simulink model "ELEC4110"  (Simulink 10.1)
settings: Solver=FixedStepDiscrete  StartTime=0.0  StopTime=200  RelTol=1e-3
PreLoadFcn:
  | qpsktxrx = commqpsktxrx_init();
InitFcn:
  | %qpsktxrx = commqpsktxrx_init();
  | ELEC4110_Init;
values from neighbouring files (symbols this model uses):
  H_CSIR = H_static    [ELEC4110_Init.m]
  maxTOffset = 50    [ELEC4110_Init.m]
  numInterpRx = 8    [ELEC4110_Init.m]
  numSampPerSym = RxSampleSize / TotalFrameSize    [ELEC4110_Init.m]
  PreambleSize = losmimo.SeqLength    [ELEC4110_Init.m]
  TotalDataPreambleSize = losmimo.DataLength/log2(losmimo.M) + losmimo.SeqLength    [ELEC4110_Init.m]
  TxPreamble = [losmimo.PNSymbols; losmimo.PNSymbols1; losmimo.PNSymbols2; losmimo.PNSymbols3; losmimo.PNSymbols4; losmimo.PNSymbols5; losmimo.PNSymbols6; losmimo.PNSymbols7]    [ELEC4110_Init.m]
undefined symbols (not defined in the file or in its folder): losmimo
libraries: commfilt2 x4, commsink2 x2, commdigbbndam3 x2, commchan3 x1, dspsrcs4 x1, dspsigops x1
Description:
  | QPSK Transmitter and Receiver.
  | 
  | This model shows the implementation of a QPSK transmitter and receiver.
settings Model: FPTRunName=Active  Creator=The MathWorks, Inc.  LastModifiedBy=eeknlau
settings DataIOCC: LimitDataPoints=on  SaveOutput=off  SaveTime=off
settings OptimizationCC: BooleanDataType=off  DefaultParameterBehavior=Inlined  ExpressionDepthLimit=2147483647  LocalBlockOutputs=off
settings DebuggingCC: AlgebraicLoopMsg=error  SolverPrmCheckMsg=warning  SingleTaskRateTransMsg=error  ParameterPrecisionLossMsg=none  AllowSymbolicDim=off  StateNameClashWarn=warning
settings HardwareCC: TargetBitPerLong=64  TargetBitPerPointer=64  TargetBitPerSizeT=64  TargetBitPerPtrDiffT=64  TargetLongLongMode=on  TargetIntDivRoundTo=Zero  TargetEndianess=LittleEndian  TargetWordSize=64  TargetHWDeviceType=Generic->MATLAB Host Computer  ProdEqTarget=off
settings GRTTargetCC: CombineOutputUpdateFcns=on  GRTInterface=off
settings ConfigComp: CovShowResultsExplorer=off  CovSFcnEnable=off
settings SimEventsCC: propDiagStatOutput=1  propPreventDuplicateEvents=0

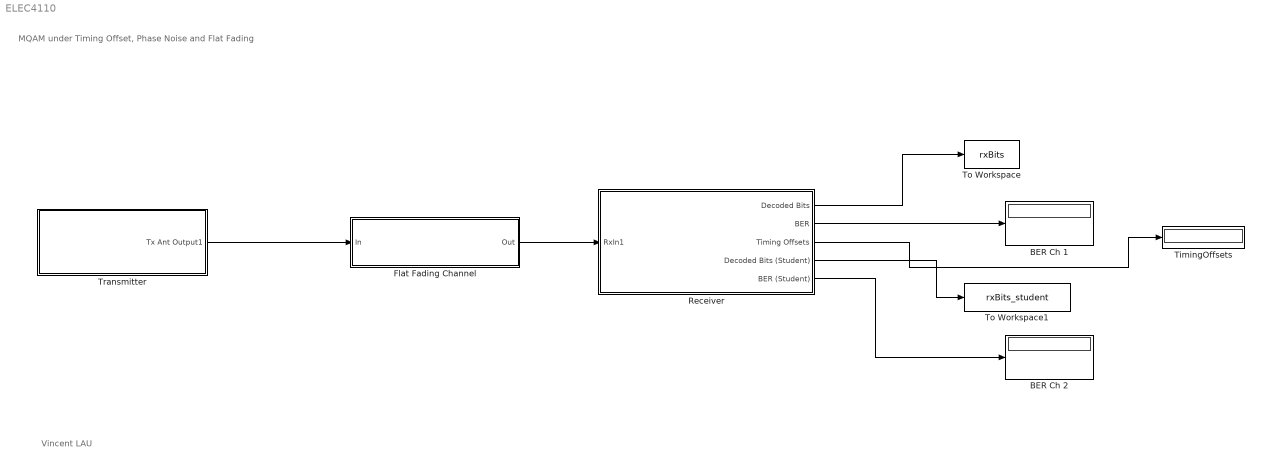
== system ELEC4110 ==
  note: MQAM under Timing Offset, Phase Noise and Flat Fading
  note: Vincent LAU
  BER Ch 1 : Display
  BER Ch 2 : Display
  Flat Fading Channel : Subsystem
      mask Display: disp('Flat Fading Channel');
  Receiver : Subsystem
      mask Display: disp('MQAM Receiver with Timing Sync\n Channel Equalization & Demod\n')
  TimingOffsets : Display
  To Workspace : ToWorkspace  VariableName=rxBits  SaveFormat=Structure  SampleTime=-1
  To Workspace1 : ToWorkspace  VariableName=rxBits_student  SaveFormat=Structure  SampleTime=-1
  Transmitter : Subsystem
      mask Display: disp('Transmitter with\n Phase Noise\n & Timing Offsets')
  wires:
  Transmitter/1(Tx Ant Output1) -> Flat Fading Channel/1(In)
  Flat Fading Channel/1(Out) -> Receiver/1(RxIn1)
  Receiver/2(BER) -> BER Ch 1/1
  Receiver/1(Decoded Bits) -> To Workspace/1
  Receiver/3("Timing Offsets ") -> TimingOffsets/1
  Receiver/4(Decoded Bits (Student)) -> To Workspace1/1
  Receiver/5(BER (Student)) -> BER Ch 2/1

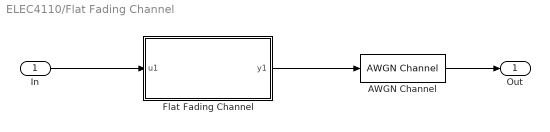
== system ELEC4110/Flat Fading Channel ==
  In : Inport
  AWGN Channel : commchan3/AWGN Channel  InputProcessing=Columns as channels (frame based)  seed=67  noiseMode="Signal to noise ratio  (SNR)"  EbNodB=10  EsNodB=10  SNRdB=RxSNRdB  bitsPerSym=1  Ps=1  Tsym=1  variance=1
  Flat Fading Channel : MATLAB Function  TreatAsAtomicUnit=on
  Out : Outport  VectorParamsAs1DForOutWhenUnconnected=off
  wires:
  In/1 -> Flat Fading Channel/1(u1)
  Flat Fading Channel/1(y1) -> AWGN Channel/1
  AWGN Channel/1 -> Out/1

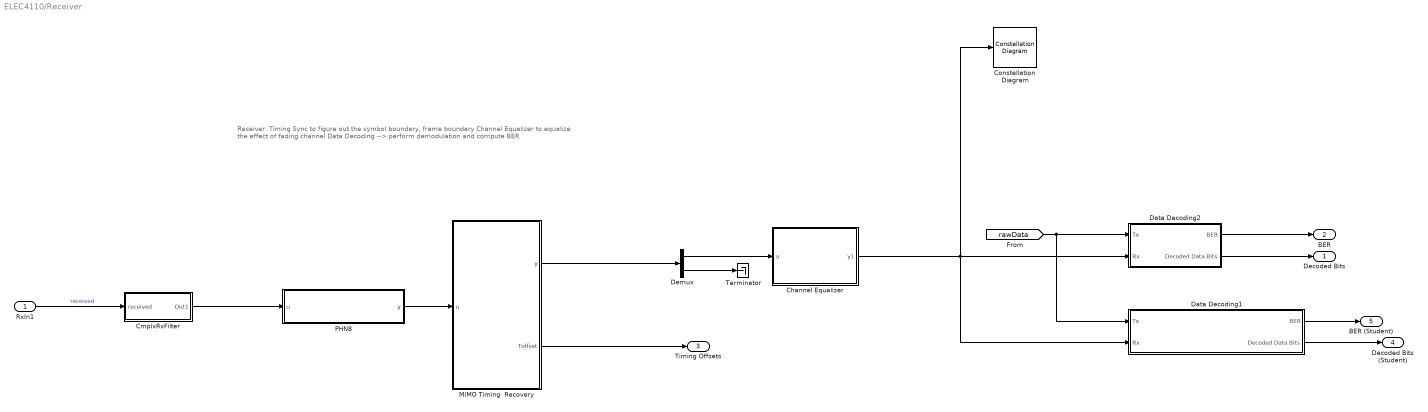
== system ELEC4110/Receiver ==
  note: Receiver: Timing Sync to figure out the symbol boundary, frame boundary
      | Channel Equalizer to equalize the effect of fading channel
      | Data Decoding --> perform demodulation and compute BER
  RxIn1 : Inport
  Channel Equalizer : MATLAB Function  TreatAsAtomicUnit=on
  CmplxRxFilter : Subsystem
  Constellation Diagram : ConstellationDiagram
  Data Decoding1 : Subsystem
      mask Display: disp('Student''s Data Decoding');
  Data Decoding2 : Subsystem
      mask Display: disp('Data Decoding');
  Demux : Demux  Outputs=[TotalDataPreambleSize -1]
  MIMO Timing  Recovery : MATLAB Function  TreatAsAtomicUnit=on
  PHN8 : MATLAB Function  TreatAsAtomicUnit=on
  Terminator : Terminator
  Decoded Bits : Outport  VectorParamsAs1DForOutWhenUnconnected=off
  BER : Outport  Port=2  VectorParamsAs1DForOutWhenUnconnected=off
  "Timing Offsets " : Outport  Port=3  VectorParamsAs1DForOutWhenUnconnected=off
  Decoded Bits (Student) : Outport  Port=4  VectorParamsAs1DForOutWhenUnconnected=off
  BER (Student) : Outport  Port=5  VectorParamsAs1DForOutWhenUnconnected=off
  wires:
  RxIn1/1 -> CmplxRxFilter/1(received)  "received"
  PHN8/1(y) -> MIMO Timing  Recovery/1(u)
  CmplxRxFilter/1(Out1) -> PHN8/1(u)
  Data Decoding2/2(Decoded Data Bits) -> Decoded Bits/1
  Channel Equalizer/1(y1) -> Data Decoding1/2(Rx), Data Decoding2/2(Rx), Constellation Diagram/1
  Data Decoding2/1(BER) -> BER/1
  MIMO Timing  Recovery/1(y) -> Demux/1
  Demux/1 -> Channel Equalizer/1(u)
  [rawData] -> Data Decoding1/1(Tx), Data Decoding2/1(Tx)
  Demux/2 -> Terminator/1
  MIMO Timing  Recovery/2(Toffset) -> "Timing Offsets "/1
  Data Decoding1/1(BER) -> BER (Student)/1
  Data Decoding1/2(Decoded Data Bits) -> Decoded Bits (Student)/1

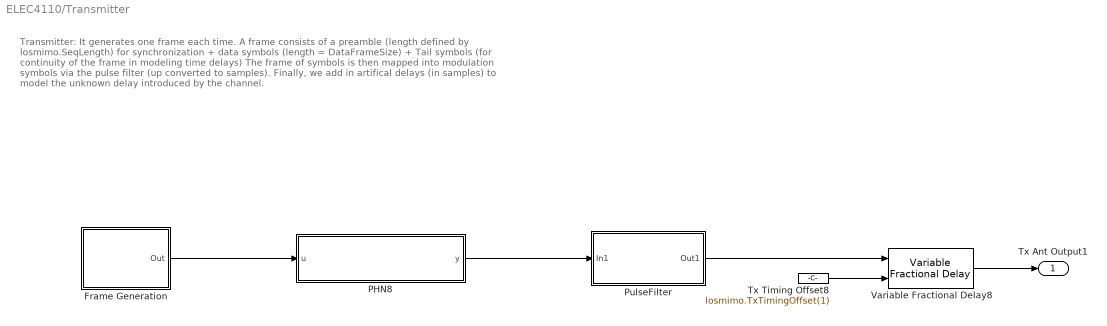
== system ELEC4110/Transmitter ==
  note: Transmitter: It generates one frame each time. A frame consists of
      |  a preamble (length defined by losmimo.SeqLength) for synchronization +
      |  data symbols (length = DataFrameSize) +
      | Tail symbols (for continuity of the frame in modeling time delays)
      | The frame of symbols is then mapped into modulation symbols via the pulse filter (up converted to samples).
      | Finally, we add in artifical delays (in samples) to model the unknown delay
      | introduced by the channel.
  Frame Generation : Subsystem
      mask Display: disp('Frame Generation')
  PHN8 : MATLAB Function  TreatAsAtomicUnit=on
  PulseFilter : Subsystem
  Tx Timing Offset8 : Constant  Value=losmimo.TxTimingOffset(1)
  Variable Fractional Delay8 : dspsigops/Variable Fractional Delay  mode=OBSOLETE  modeActive=Farrow  L=4  FarrowL=3  R=50  alpha=1  dmax=20  InputProcessing=Columns as channels (frame based)  ic=0  noDFT=off  fallbackFIR=Clip to the minimum value necessary for centered kernel  fallbackFarrow=Clip to the minimum value necessary for centered kernel  roundingMode=Zero  overflowMode=off
      settings: SourceProductBaseCode=DS
  Tx Ant Output1 : Outport  VectorParamsAs1DForOutWhenUnconnected=off
  wires:
  PHN8/1(y) -> PulseFilter/1(In1)
  Frame Generation/1(Out) -> PHN8/1(u)
  Tx Timing Offset8/1 -> Variable Fractional Delay8/2
  PulseFilter/1(Out1) -> Variable Fractional Delay8/1
  Variable Fractional Delay8/1 -> Tx Ant Output1/1

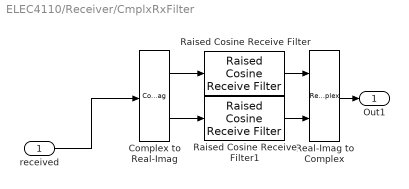
== system ELEC4110/Receiver/CmplxRxFilter ==
  received : Inport
  Complex to Real-Imag : ComplexToRealImag
  Raised Cosine Receive Filter : commfilt2/Raised Cosine Receive Filter  filtType=Square root  R=losmimo.RolloffFactor  filtSpan=losmimo.RaisedCosineFilterSpan  N=losmimo.Upsampling  downFactor=losmimo.Decimation  downOffset=0  filterGain=1  InputProcessing=Columns as channels (frame based)  RateOptions=Enforce single-rate processing  framing=Mute  checkCoeff=off  variableName=rcRxFilt  currentFiltSpan=10  D=5  inputOffset=0  sampMode=Mute  saveAsFlag=0  rateMode=Downsampling  checkGain=Normalized  launchFVT=on  roundingMode=Floor  overflowMode=off  coeffDataTypeStr=Inherit: Same word length as input  coeffMin=[]  coeffMax=[]  coeffLastDataTypeStr=Inherit: Same word length as input  accumDataTypeStr=Inherit: Same as product output  accumLastDataTypeStr=Inherit: Same as product output  outputDataTypeStr=Inherit: Same as accumulator  outputMin=[]  outputMax=[]  outputLastDataTypeStr=Inherit: Same as accumulator
  Raised Cosine Receive Filter1 : commfilt2/Raised Cosine Receive Filter  filtType=Square root  R=losmimo.RolloffFactor  filtSpan=losmimo.RaisedCosineFilterSpan  N=losmimo.Upsampling  downFactor=losmimo.Decimation  downOffset=0  filterGain=1  InputProcessing=Columns as channels (frame based)  RateOptions=Enforce single-rate processing  framing=Mute  checkCoeff=off  variableName=rcRxFilt1  currentFiltSpan=10  D=5  inputOffset=0  sampMode=Mute  saveAsFlag=0  rateMode=Downsampling  checkGain=Normalized  launchFVT=on  roundingMode=Floor  overflowMode=off  coeffDataTypeStr=Inherit: Same word length as input  coeffMin=[]  coeffMax=[]  coeffLastDataTypeStr=Inherit: Same word length as input  accumDataTypeStr=Inherit: Same as product output  accumLastDataTypeStr=Inherit: Same as product output  outputDataTypeStr=Inherit: Same as accumulator  outputMin=[]  outputMax=[]  outputLastDataTypeStr=Inherit: Same as accumulator
  Real-Imag to Complex : RealImagToComplex
  Out1 : Outport  VectorParamsAs1DForOutWhenUnconnected=off
  wires:
  Raised Cosine Receive Filter1/1 -> Real-Imag to Complex/2
  Complex to Real-Imag/1 -> Raised Cosine Receive Filter/1
  received/1 -> Complex to Real-Imag/1
  Real-Imag to Complex/1 -> Out1/1
  Raised Cosine Receive Filter/1 -> Real-Imag to Complex/1
  Complex to Real-Imag/2 -> Raised Cosine Receive Filter1/1

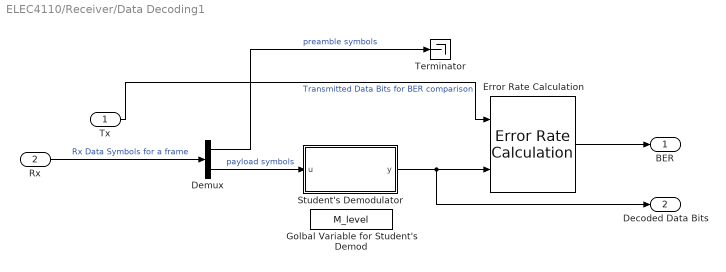
== system ELEC4110/Receiver/Data Decoding1 ==
  Tx : Inport
  Rx : Inport  Port=2
  Demux : Demux  Outputs=[[PreambleSize -1]]
  Error Rate Calculation : commsink2/Error Rate Calculation  N=0  st_delay=0  cp_mode=Entire frame  subframe=[]  PMode=Port  WsName=ErrorVec  RsMode2=off  stop=off  numErr=100  maxBits=1e6
  Golbal Variable for Student's Demod : DataStoreMemory  DataStoreName=M_level  ReadBeforeWriteMsg=warning  WriteAfterWriteMsg=warning  WriteAfterReadMsg=warning  ShowAdditionalParam=off  OutDataTypeStr=int16
  Student's Demodulator : MATLAB Function  TreatAsAtomicUnit=on
  Terminator : Terminator
  BER : Outport  VectorParamsAs1DForOutWhenUnconnected=off
  Decoded Data Bits : Outport  Port=2  VectorParamsAs1DForOutWhenUnconnected=off
  wires:
  Error Rate Calculation/1 -> BER/1
  Student's Demodulator/1(y) -> Decoded Data Bits/1, Error Rate Calculation/2
  Demux/1 -> Terminator/1  "preamble symbols"
  Rx/1 -> Demux/1  "Rx Data Symbols for a frame"
  Demux/2 -> Student's Demodulator/1(u)  "payload symbols"
  Tx/1 -> Error Rate Calculation/1  "Transmitted Data Bits for BER comparison"

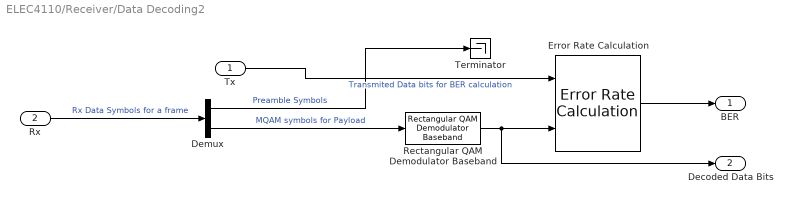
== system ELEC4110/Receiver/Data Decoding2 ==
  Tx : Inport
  Rx : Inport  Port=2
  Demux : Demux  Outputs=[[PreambleSize -1]]
  Error Rate Calculation : commsink2/Error Rate Calculation  N=0  st_delay=0  cp_mode=Entire frame  subframe=[]  PMode=Port  WsName=ErrorVec  RsMode2=off  stop=off  numErr=100  maxBits=1e6
  Rectangular QAM Demodulator Baseband : commdigbbndam3/Rectangular QAM Demodulator Baseband  M=losmimo.M  OutType=Bit  DecType=Hard decision  VarSource=Dialog  Variance=1  Dec=Gray  Mapping=[0:15]  PowType=Average Power  MinDist=2  AvgPow=1  PeakPow=1  Ph=0  outDtype1=Inherit via internal rule  outDtype2=Inherit via internal rule  derotateFactorWordLen=16  derotateFactorDataTypeStr=Inherit: Same word length as input  derotateFactorLastDataTypeStr=Inherit: Same word length as input  denormFactorWordLen=16  denormFactorDataTypeStr=Inherit: Same word length as input  denormFactorLastDataTypeStr=Inherit: Same word length as input  prodOutWordLen=32  prodOutOverflowMode=Wrap  prodOutRoundingMode=Floor  prodOutOvFlMode=off  prodOutOvFlModeLastStrValue=off  sumWordLen=32
  Terminator : Terminator
  BER : Outport  VectorParamsAs1DForOutWhenUnconnected=off
  Decoded Data Bits : Outport  Port=2  VectorParamsAs1DForOutWhenUnconnected=off
  wires:
  Error Rate Calculation/1 -> BER/1
  Rectangular QAM Demodulator Baseband/1 -> Decoded Data Bits/1, Error Rate Calculation/2
  Demux/1 -> Terminator/1  "Preamble Symbols"
  Rx/1 -> Demux/1  "Rx Data Symbols for a frame"
  Demux/2 -> Rectangular QAM Demodulator Baseband/1  "MQAM symbols for Payload"
  Tx/1 -> Error Rate Calculation/1  "Transmited Data bits for BER calculation"

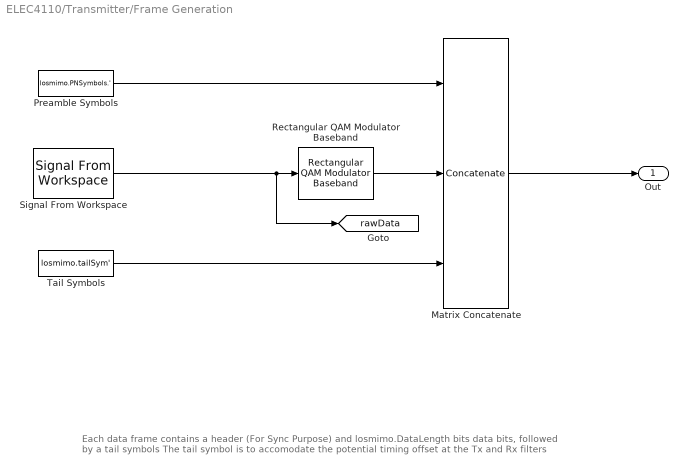
== system ELEC4110/Transmitter/Frame Generation ==
  note: Each data frame contains a header (For Sync Purpose) and losmimo.DataLength bits data bits,
      | followed by a tail symbols The tail symbol is to accomodate the potential timing offset at the Tx and Rx filters
  Matrix Concatenate : Concatenate  NumInputs=3  Mode=Multidimensional array
  Preamble Symbols : Constant  Value=losmimo.PNSymbols.'  VectorParams1D=off  OutDataTypeStr=double
  Rectangular QAM Modulator Baseband : commdigbbndam3/Rectangular QAM Modulator Baseband  M=losmimo.M  InType=Bit  Enc=Gray  Mapping=[0:15]  PowType=Average Power  MinDist=2  AvgPow=1  PeakPow=1  Ph=0  outDtype=double  outWordLen=16  outUDDataType=sfix(16)  outFracLenMode=Best precision  outFracLen=15  outDataTypeStr=double  outLastDataTypeStr=double
  Signal From Workspace : dspsrcs4/Signal From Workspace  X=losmimo.sBit  Ts=1/losmimo.DataLength*losmimo.FrameTime  nsamps=losmimo.DataLength  OutputAfterFinalValue=Cyclic repetition  ignoreOrWarnInputAndFrameLengths=off  OutputFrames=off
  Tail Symbols : Constant  Value=losmimo.tailSym'  VectorParams1D=off  OutDataTypeStr=double
  Out : Outport  VectorParamsAs1DForOutWhenUnconnected=off
  tag scope: rawData=global
  wires:
  Signal From Workspace/1 -> [rawData], Rectangular QAM Modulator Baseband/1
  Rectangular QAM Modulator Baseband/1 -> Matrix Concatenate/2
  Matrix Concatenate/1 -> Out/1
  Preamble Symbols/1 -> Matrix Concatenate/1
  Tail Symbols/1 -> Matrix Concatenate/3

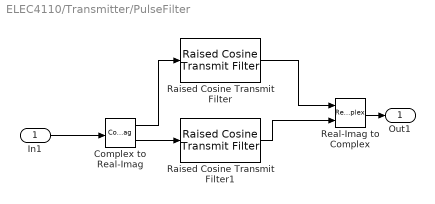
== system ELEC4110/Transmitter/PulseFilter ==
  In1 : Inport
  Complex to Real-Imag : ComplexToRealImag
  Raised Cosine Transmit Filter : commfilt2/Raised Cosine Transmit Filter  filtType=Square root  R=losmimo.RolloffFactor  filtSpan=losmimo.RaisedCosineFilterSpan  N=losmimo.Upsampling  filterGain=1  InputProcessing=Columns as channels (frame based)  RateOptions=Enforce single-rate processing  framing=Mute  checkCoeff=off  variableName=rcTxFilt1  checkGain=Normalized  sampMode=Mute  saveAsFlag=0  currentFiltSpan=10  D=5  launchFVT=on  roundingMode=Floor  overflowMode=off  coeffDataTypeStr=Inherit: Same word length as input  coeffMin=[]  coeffMax=[]  coeffLastDataTypeStr=Inherit: Same word length as input  outputDataTypeStr=Inherit: Same as accumulator  outputMin=[]  outputMax=[]  outputLastDataTypeStr=Inherit: Same as accumulator
  Raised Cosine Transmit Filter1 : commfilt2/Raised Cosine Transmit Filter  filtType=Square root  R=losmimo.RolloffFactor  filtSpan=losmimo.RaisedCosineFilterSpan  N=losmimo.Upsampling  filterGain=1  InputProcessing=Columns as channels (frame based)  RateOptions=Enforce single-rate processing  framing=Mute  checkCoeff=off  variableName=rcTxFilt1  checkGain=Normalized  sampMode=Mute  saveAsFlag=0  currentFiltSpan=10  D=5  launchFVT=on  roundingMode=Floor  overflowMode=off  coeffDataTypeStr=Inherit: Same word length as input  coeffMin=[]  coeffMax=[]  coeffLastDataTypeStr=Inherit: Same word length as input  outputDataTypeStr=Inherit: Same as accumulator  outputMin=[]  outputMax=[]  outputLastDataTypeStr=Inherit: Same as accumulator
  Real-Imag to Complex : RealImagToComplex
  Out1 : Outport  VectorParamsAs1DForOutWhenUnconnected=off
  wires:
  Complex to Real-Imag/1 -> Raised Cosine Transmit Filter/1
  Real-Imag to Complex/1 -> Out1/1
  Raised Cosine Transmit Filter1/1 -> Real-Imag to Complex/2
  In1/1 -> Complex to Real-Imag/1
  Raised Cosine Transmit Filter/1 -> Real-Imag to Complex/1
  Complex to Real-Imag/2 -> Raised Cosine Transmit Filter1/1

== matlab function Receiver/Data Decoding1/Student's Demodulator ==
  data: u input double; y output double [..17400]; M_level data_store_memory double
function y = MQAM_Demod(u)

global M_level
%global numDataBits;
NumSym = length(u); % Number of received symbols
% Put your demodulator design here



y = randi([0,1],17400,1); % fix output size to total # of Tx bits
%y = randi([0,1],log2(M_level)*NumSym,1);  % dummy outputs (assuming 16 QAM)
% Write your output

== matlab function Transmitter/PHN8 ==
  data: u input double size=TotalFrameSize; y output double size=TotalFrameSize; sigma_PHN parameter double
function y = PhNoiseGen(u,sigma_PHN)
% sigma_PHN = std deviation of the PHN (defined as workspace variable)
% in degree.
% Please implement the PHN generator using Wiener model as in that paper
% (in email). 



y = u;

== matlab function Receiver/PHN8 ==
  data: u input double; y output double; sigma_PHN parameter double
function y = PhNoiseGen(u,sigma_PHN)
% sigma_PHN = std deviation of the PHN (defined as workspace variable)
% in degree.
% Please implement the PHN generator using Wiener model as in that paper
% (in email). 



y = u;

== matlab function Flat Fading Channel/Flat Fading Channel ==
  data: u1 input double size=TxSampleSize; y1 output double size=TxSampleSize; H_static parameter double
function y1  = Fading_Ch(u1, H_static)
% Input: u1 = tx samples from 1 Tx antennas
% Output: y1 = rx samples after fading channel 
% H_static = static fading channel [Complex] (Compute Offline and initialize in the ELEC4110_Init.m 


y1 = H_static*(u1);  % y1 is the channel outputs (8 x Tsize)

== matlab function Receiver/Channel Equalizer ==
  data: u input double; y1 output double; H_CSIR parameter double; PreambleSize parameter double
function y1  = ChannelEqualizer(u,H_CSIR, PreambleSize)
% inputs u = 8Len x 1 column vectors (concatenated samples from 8 streams). 
% parameter = CSIR (1x1 estimate of channel fading H)
% Compute the Decorrelator 


Tsize = length(u);
%[U,S,V] = svd(H_CSIR);
input = reshape(u,[Tsize,1]).'; %input = 8 x numSamp
tIdx = [PreambleSize+1:Tsize];
r = (H_CSIR'/abs(H_CSIR)^2)*input(:,tIdx);   % equalizer output r =  numSamp (only apply to payload symbols)

% Equalize the H per stream after Decorrelation so that the rx
% constellation is aligned with the standard constellation for demod

% For each stream, normalize w.r.t channel gain (SVD e-values) so that the
% demodulation constellation will match the Tx constellation
%for i = 1:8
%    r(i,:) = r(i,:)./S(i,i);
%end
y1 = input(1,:).';
y1(tIdx) = r(1,:).';

== matlab function Receiver/MIMO Timing Recovery ==
  data: u input double; y output double; TxPreamble parameter double; numSampPerSym parameter double; TotalDataPreambleSize parameter double; numInterpRx parameter double; maxTOffset parameter double; Toffset output double
function [y,Toffset]  = Timing_Sync(u,TxPreamble, numSampPerSym, TotalDataPreambleSize, numInterpRx,maxTOffset)

% Perform Timing Sync
% u Input samples (T x 1)
% y, ...... Output symbols (synchronized to 1 sample (optimally sampled)
% % Tx Preambles = Np
% numSampPerSym = # of samples per symbol in the input stream
% TotalFrameSize = # of symbols per frame in the outputs
% numInterpRx = interpolation factor within timing recovery.
% maxTOffset = max # of timing offset at Tx (# of symbols)


inSize = length(u);
y=u;    % set the size of y = that of u so that the block will have fixed size input and output
Toffset = 0;

% separate the u into 8 input streams (input = inSize x 8)
input = u;
%input = (W_decor*(input0.')).';


% Interpoluation for the input samples 
PLen = length(TxPreamble(1,:));  % num of symbols in a preamble
PIntv = numSampPerSym*numInterpRx;  % number of interpolated samples per symbol
Tdepth = maxTOffset * PIntv;  % max timing offset in number of interpolated samples
xt = [1:numInterpRx:inSize*numInterpRx];
xq = [1:inSize*numInterpRx];
interp_u = zeros(inSize*numInterpRx,1)+1i*zeros(inSize*numInterpRx,1);

interp_u(:,1) = interp1(xt,real(input(:,1)),xq,'spline')+1i*interp1(xt,imag(input(:,1)),xq,'spline'); % generate interpolated samples at PIntv times of the input

% search for preamble in the interp samples
baseIdx = [0:PIntv:PLen*PIntv-1]; % base index for samples used to compute timing metric 
baseIdx2 = [0:PIntv:(PIntv*TotalDataPreambleSize -1)];   % base index for taking out samples from interpolated samples to form output frame
metric = zeros(1,Tdepth);

    for t=1:Tdepth
        % compute timing metric for 8 data streams
        metric(1,t) = compputeTimingMetric(interp_u(baseIdx+t,1),TxPreamble(1,:).');
%         TimingMetric(n,t) = (1-alpha)*TimingMetric(n,t) + alpha*metric;
    end

maxVal = zeros(1,1);
maxtIdx = zeros(1,1);
% search for max metric over t for each stream
temp = zeros(TotalDataPreambleSize,1)+1i*zeros(TotalDataPreambleSize,1);
    [maxVal(1), maxtIdx(1)] = max(metric(1,:));

    % maxtIdx corresponds to the sample index of the frame start
    tOutIdx = maxtIdx(1) + baseIdx2;
    temp(:,1) = interp_u(tOutIdx,1);
y(1:TotalDataPreambleSize) = reshape(temp,[TotalDataPreambleSize,1]);
Toffset = maxtIdx;
